simulink library "Lidar_IdealWind_16b"  (Simulink 8.8)
settings: Solver=VariableStepAuto  StartTime=0.0  StopTime=10.0  RelTol=1e-3
undefined symbols (not defined in the file): Atmosphere, CRM, IdealWind, LIDAR, SimConfig, WindReconstruction
libraries: simulink x1
settings Model: SuppressorTable="22 serialization::archive 15 0 6 0 0 1 8 0 0 0 0 6 0 0 1 0 93 Lidar_IdealWind_16b/Lidar_IdealWind/TriggerEstimation/Repeating Sequence Stair/LimitedCounter 0 6 0 0 2 8 0 0 0 0 6 41 Simulink:DataType:WarningOverFlowDetected 0 0 0 6 0  0  0 0 0 0 8 20160608 0 0 0 15 23 17 0 1 40 SimulinkFixedPoint:util:Overflowoccurred 0 0 0  0  8 20160608 0 15 23 17 0 1"  Creator=cava_da  LastModifiedBy=cava_da

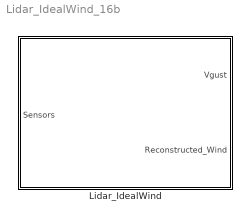
== system Lidar_IdealWind_16b ==
  Lidar_IdealWind : Subsystem

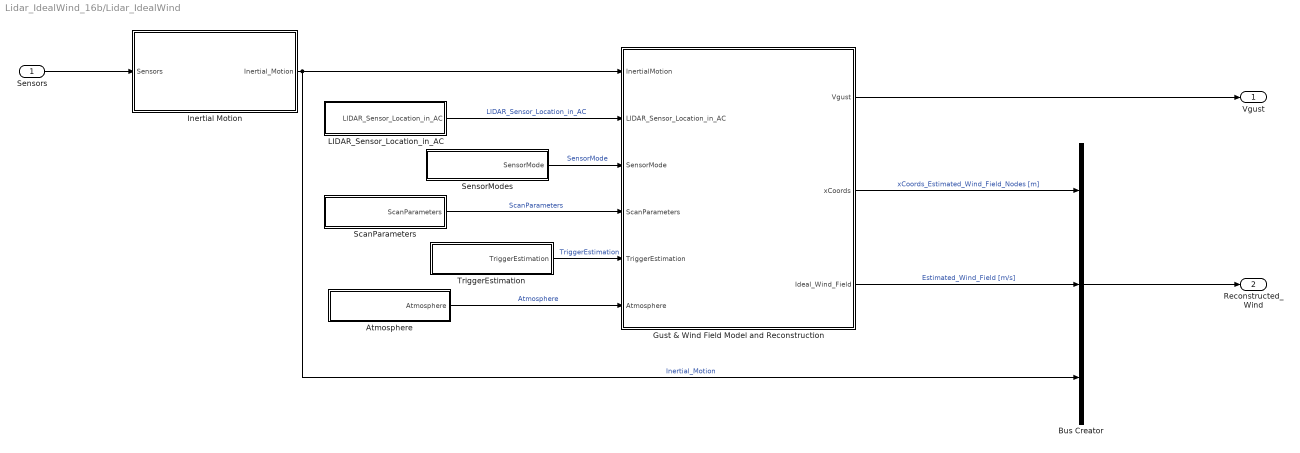
== system Lidar_IdealWind_16b/Lidar_IdealWind ==
  Sensors : Inport
  Atmosphere : Subsystem
  Bus Creator : BusCreator  Inputs=3
  Gust & Wind Field Model and Reconstruction : Subsystem
  Inertial Motion : Subsystem
  LIDAR_Sensor_Location_in_AC : Subsystem
  ScanParameters : Subsystem
  SensorModes : Subsystem
  TriggerEstimation : Subsystem
  Vgust : Outport
  Reconstructed_Wind : Outport  Port=2
  wires:
  Bus Creator/1 -> Reconstructed_Wind/1
  Atmosphere/1(Atmosphere) -> Gust & Wind Field Model and Reconstruction/6(Atmosphere)  "Atmosphere"
  Gust & Wind Field Model and Reconstruction/1(Vgust) -> Vgust/1
  Gust & Wind Field Model and Reconstruction/3(Ideal_Wind_Field) -> Bus Creator/2  "Estimated_Wind_Field [m/s]"
  Gust & Wind Field Model and Reconstruction/2(xCoords) -> Bus Creator/1  "xCoords_Estimated_Wind_Field_Nodes [m]"
  Inertial Motion/1(Inertial_Motion) -> Gust & Wind Field Model and Reconstruction/1(InertialMotion), Bus Creator/3  "Inertial_Motion"
  TriggerEstimation/1(TriggerEstimation) -> Gust & Wind Field Model and Reconstruction/5(TriggerEstimation)  "TriggerEstimation"
  ScanParameters/1(ScanParameters) -> Gust & Wind Field Model and Reconstruction/4(ScanParameters)  "ScanParameters"
  SensorModes/1(SensorMode) -> Gust & Wind Field Model and Reconstruction/3(SensorMode)  "SensorMode"
  LIDAR_Sensor_Location_in_AC/1(LIDAR_Sensor_Location_in_AC) -> Gust & Wind Field Model and Reconstruction/2(LIDAR_Sensor_Location_in_AC)  "LIDAR_Sensor_Location_in_AC"
  Sensors/1 -> Inertial Motion/1(Sensors)

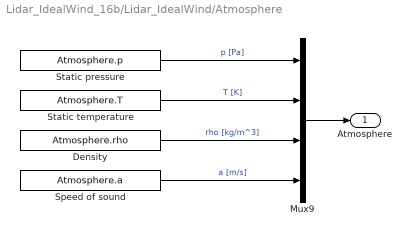
== system Lidar_IdealWind_16b/Lidar_IdealWind/Atmosphere ==
  Density : Constant  Value=Atmosphere.rho
  Mux9 : Mux
  Speed of sound : Constant  Value=Atmosphere.a
  Static pressure : Constant  Value=Atmosphere.p
  Static temperature : Constant  Value=Atmosphere.T
  Atmosphere : Outport
  wires:
  Speed of sound/1 -> Mux9/4  "a [m/s]"
  Density/1 -> Mux9/3  "rho [kg/m^3]"
  Static temperature/1 -> Mux9/2  "T [K]"
  Static pressure/1 -> Mux9/1  "p [Pa]"
  Mux9/1 -> Atmosphere/1

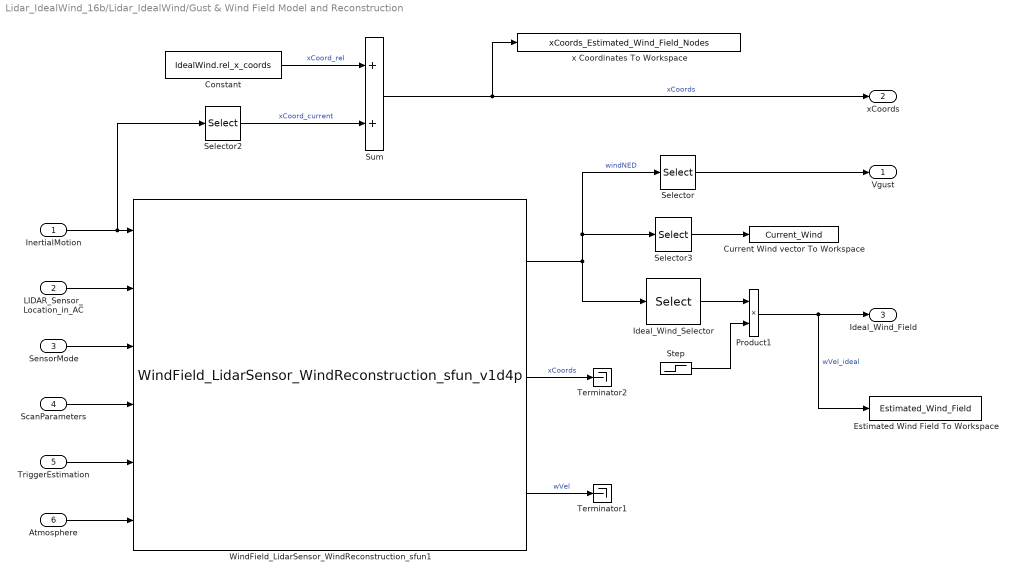
== system Lidar_IdealWind_16b/Lidar_IdealWind/Gust & Wind Field Model and Reconstruction ==
  InertialMotion : Inport
  LIDAR_Sensor_Location_in_AC : Inport  Port=2
  SensorMode : Inport  Port=3
  ScanParameters : Inport  Port=4
  TriggerEstimation : Inport  Port=5
  Atmosphere : Inport  Port=6
  Constant : Constant  Value=IdealWind.rel_x_coords
  Current Wind vector To Workspace : ToWorkspace  VariableName=Current_Wind  SaveFormat=Structure  SampleTime=-1
  Estimated Wind Field To Workspace : ToWorkspace  VariableName=Estimated_Wind_Field  SaveFormat=Structure With Time  SampleTime=-1
      settings: Decimation=SimConfig.Logging.DecimationFactor
  Ideal_Wind_Selector : Selector  IndexOptions=Starting index (dialog)  Indices=4  OutputSizes=IdealWind.n_nodes
  Product1 : Product  RndMeth=Zero
  Selector : Selector  IndexOptions=Index vector (dialog)  Indices=3  OutputSizes=1
  Selector2 : Selector  IndexOptions=Index vector (dialog)  Indices=1  OutputSizes=1
  Selector3 : Selector  IndexOptions=Index vector (dialog)  Indices=1:3  OutputSizes=1
  Step : Step  Time=WindReconstruction.StartEstimationTime  SampleTime=0
  Sum : Sum
  Terminator1 : Terminator
  Terminator2 : Terminator
  WindField_LidarSensor_WindReconstruction_sfun1 : S-Function  FunctionName=WindField_LidarSensor_WindReconstruction_sfun_v1d4p  Parameters=Atmosphere,LIDAR,WindReconstruction  SFunctionDeploymentMode=off  EnableBusSupport=off  mask(Direct detection wind lidar and wind reconstruction (s-function)){}
      mask help:
      | This s-function incorporates the model of a direct detection Doppler wind lidar coupled with a wind reconstruction algorithm based on maximum likelihood estimation. It also serves as the interface between the included wind model and the encompassing aeroelastic aircraft model via the configurable wind output (output port 1).
      | The lidar model and the wind reconstruction algorithm are technically independent modules, but are implemented in the same s-function for performance reasons.
      |
      | Output port 1: wind output, configurable via the parameter Atmosphere.WindConfig
      | Output port 2: x-coordinates of the estimation nodes in geodetic frame and in meters
      | Output port 3: vertical wind speed at the estimation nodes in m/s
      |
      | Output ports 2 and 3 are only updated when a new estimation was triggered via input port 5.
      |
      | Detailed documentation is found under: https://github.com/dlr-ft-gla/GLA-Benchmark/wiki
      |
      |
      |
      | (c) Copyright 2021 DLR e. V.
      |
      | Institute of Flight Systems, 38108 Braunschweig, Germany.
      | Institute of Atmospheric Physics, 82234 Wessling, Germany.
      |
      | Authors:
      | Daniel Kiehn (daniel.kiehn@dlr.de)
      | Nicolas Fezans (nicolas.fezans@dlr.de)
      | Patrick Vrancken (patrick.vrancken@dlr.de)
      |
      | Block and underlying s-function released under CC-BY-ND 4.0 license.
      | https://creativecommons.org/licenses/by-nd/4.0/
      mask Help: For help, please refer to the online documentation of the CRM benchmark model: <a href="matlab: web('https://github.com/dlr-ft-gla/GLA-Benchmark/wiki')">https://github.com/dlr-ft-gla/GLA-Benchmark/wiki</a>.
      mask Display:
      | port_label('input', 1, 'Inertial motion');
      | port_label('input', 2, 'Sensor location in AC');
      | port_label('input', 3, 'Sensor mode');
      | port_label('input', 4, 'Scan parameters');
      | port_label('input', 5, 'Estimation trigger');
      | port_label('input', 6, 'Atmosphere');
      | 
      | port_label('output', 1, 'AC wind inputs');
      | port_label('output', 2, 'x coordinates');
      | port_label('output', 3, 'Estimated wind');
      | 
      | image(imread('DLR_Logo.jpg'),[180,10,81,68])
      | 
      | disp(['DIRECT DETECTION WIND LIDAR\n',...
      | '& WIND RECONSTRUCTION ALGORITHM\n\n\n\n',...
      | '(c) Copyright 2021 DLR e. V.\n\n',...
      | 'Institute of Flight Systems\n',...
      | 'Institute of Atmospheric Physics\n\n',...
      | 'Authors:\n',...
      | 'Daniel Kiehn (daniel.kiehn@dlr.de)\n',...
      | 'Nicolas Fezans (nicolas.fezans@dlr.de)\n',...
      | 'Patrick Vrancken (patrick.vrancken@dlr.de)\n\n\n',...
      | 'Block and underlying s-function\n',...
      | 'released under CC-BY-ND 4.0 license.'])
  x Coordinates To Workspace : ToWorkspace  VariableName=xCoords_Estimated_Wind_Field_Nodes  SaveFormat=Structure With Time  SampleTime=-1
      settings: Decimation=SimConfig.Logging.DecimationFactor
  Vgust : Outport
  xCoords : Outport  Port=2
  Ideal_Wind_Field : Outport  Port=3
  wires:
  Atmosphere/1 -> WindField_LidarSensor_WindReconstruction_sfun1/6
  Selector/1 -> Vgust/1
  TriggerEstimation/1 -> WindField_LidarSensor_WindReconstruction_sfun1/5
  ScanParameters/1 -> WindField_LidarSensor_WindReconstruction_sfun1/4
  SensorMode/1 -> WindField_LidarSensor_WindReconstruction_sfun1/3
  LIDAR_Sensor_Location_in_AC/1 -> WindField_LidarSensor_WindReconstruction_sfun1/2
  InertialMotion/1 -> Selector2/1, WindField_LidarSensor_WindReconstruction_sfun1/1
  WindField_LidarSensor_WindReconstruction_sfun1/2 -> Terminator2/1  "xCoords"
  WindField_LidarSensor_WindReconstruction_sfun1/3 -> Terminator1/1  "wVel"
  Selector2/1 -> Sum/2  "xCoord_current"
  Constant/1 -> Sum/1  "xCoord_rel"
  Sum/1 -> x Coordinates To Workspace/1, xCoords/1  "xCoords"
  Selector3/1 -> Current Wind vector To Workspace/1
  WindField_LidarSensor_WindReconstruction_sfun1/1 -> Selector3/1, Selector/1, Ideal_Wind_Selector/1  "windNED"
  Step/1 -> Product1/2
  Ideal_Wind_Selector/1 -> Product1/1
  Product1/1 -> Estimated Wind Field To Workspace/1, Ideal_Wind_Field/1  "wVel_ideal"

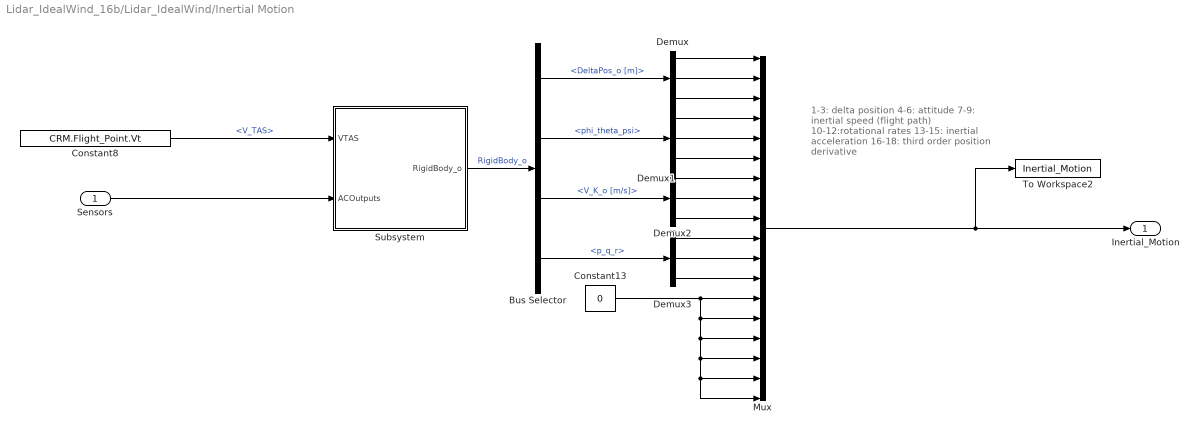
== system Lidar_IdealWind_16b/Lidar_IdealWind/Inertial Motion ==
  note: 1-3: delta position
      | 4-6: attitude
      | 7-9: inertial speed (flight path)
      | 10-12:rotational rates
      | 13-15: inertial acceleration
      | 16-18: third order position derivative
  Sensors : Inport
  Bus Selector : BusSelector  OutputSignals=DeltaPos_o [m],phi_theta_psi,V_K_o [m/s],p_q_r
  Constant13 : Constant  Value=0
  Constant8 : Constant  Value=CRM.Flight_Point.Vt
  Demux{,1..3} (4 alike) : Demux  Outputs=3
  Mux : Mux  Inputs=18
  Subsystem : Subsystem
  To Workspace2 : ToWorkspace  VariableName=Inertial_Motion  SaveFormat=Structure  SampleTime=-1
      settings: Decimation=SimConfig.Logging.DecimationFactor
  Inertial_Motion : Outport
  wires:
  Constant13/1 -> Mux/13, Mux/14, Mux/15, Mux/16, Mux/18, Mux/17
  Mux/1 -> To Workspace2/1, Inertial_Motion/1
  Constant8/1 -> Subsystem/1(VTAS)  "<V_TAS>"
  Subsystem/1(RigidBody_o) -> Bus Selector/1  "RigidBody_o"
  Sensors/1 -> Subsystem/2(ACOutputs)
  Demux3/3 -> Mux/12
  Demux3/2 -> Mux/11
  Demux3/1 -> Mux/10
  Demux2/3 -> Mux/9
  Demux2/2 -> Mux/8
  Demux2/1 -> Mux/7
  Demux1/3 -> Mux/6
  Demux1/2 -> Mux/5
  Demux1/1 -> Mux/4
  Demux/3 -> Mux/3
  Demux/2 -> Mux/2
  Demux/1 -> Mux/1
  Bus Selector/3 -> Demux2/1  "<V_K_o [m/s]>"
  Bus Selector/2 -> Demux1/1  "<phi_theta_psi>"
  Bus Selector/1 -> Demux/1  "<DeltaPos_o [m]>"
  Bus Selector/4 -> Demux3/1  "<p_q_r>"

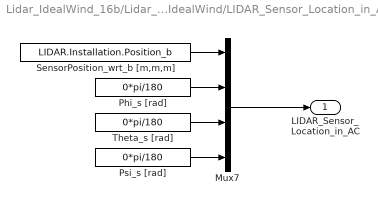
== system Lidar_IdealWind_16b/Lidar_IdealWind/LIDAR_Sensor_Location_in_AC ==
  Mux7 : Mux
  Phi_s [rad] : Constant  Value=0*pi/180
  Psi_s [rad] : Constant  Value=0*pi/180
  SensorPosition_wrt_b [m,m,m] : Constant  Value=LIDAR.Installation.Position_b
  Theta_s [rad] : Constant  Value=0*pi/180
  LIDAR_Sensor_Location_in_AC : Outport
  wires:
  Mux7/1 -> LIDAR_Sensor_Location_in_AC/1
  Psi_s [rad]/1 -> Mux7/4
  Theta_s [rad]/1 -> Mux7/3
  Phi_s [rad]/1 -> Mux7/2
  SensorPosition_wrt_b [m,m,m]/1 -> Mux7/1

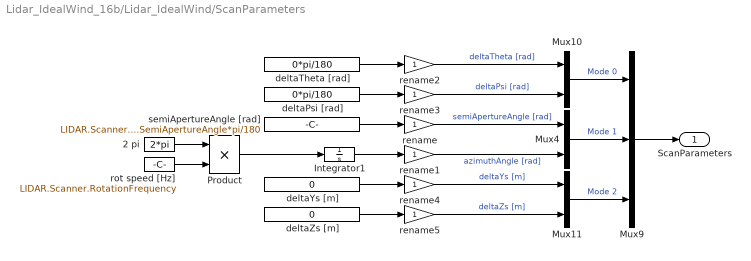
== system Lidar_IdealWind_16b/Lidar_IdealWind/ScanParameters ==
  2 pi : Constant  Value=2*pi
  Integrator1 : Integrator
  Mux10 : Mux  Inputs=2
  Mux11 : Mux  Inputs=2
  Mux4 : Mux  Inputs=2
  Mux9 : Mux  Inputs=3
  Product : Product  RndMeth=Zero
  deltaPsi [rad] : Constant  Value=0*pi/180  OutDataTypeStr=double
  deltaTheta [rad] : Constant  Value=0*pi/180  OutDataTypeStr=double
  deltaYs [m] : Constant  Value=0  OutDataTypeStr=double
  deltaZs [m] : Constant  Value=0  OutDataTypeStr=double
  rename{,1..5} (6 alike) : Gain
  rot speed [Hz] : Constant  Value=LIDAR.Scanner.RotationFrequency
  semiApertureAngle [rad] : Constant  Value=LIDAR.Scanner.SemiApertureAngle*pi/180  OutDataTypeStr=double
  ScanParameters : Outport
  wires:
  Mux9/1 -> ScanParameters/1
  Integrator1/1 -> rename1/1
  rot speed [Hz]/1 -> Product/2
  Product/1 -> Integrator1/1
  2 pi/1 -> Product/1
  semiApertureAngle [rad]/1 -> rename/1
  deltaZs [m]/1 -> rename5/1
  deltaYs [m]/1 -> rename4/1
  deltaTheta [rad]/1 -> rename2/1
  deltaPsi [rad]/1 -> rename3/1
  Mux11/1 -> Mux9/3  "Mode 2"
  Mux4/1 -> Mux9/2  "Mode 1"
  rename4/1 -> Mux11/1  "deltaYs [m]"
  rename5/1 -> Mux11/2  "deltaZs [m]"
  rename/1 -> Mux4/1  "semiApertureAngle [rad]"
  rename1/1 -> Mux4/2  "azimuthAngle [rad]"
  Mux10/1 -> Mux9/1  "Mode 0"
  rename2/1 -> Mux10/1  "deltaTheta [rad]"
  rename3/1 -> Mux10/2  "deltaPsi [rad]"

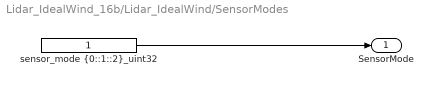
== system Lidar_IdealWind_16b/Lidar_IdealWind/SensorModes ==
  "sensor_mode {0::1::2}_uint32" : Constant  OutDataTypeStr=uint32
  SensorMode : Outport
  wires:
  "sensor_mode {0::1::2}_uint32"/1 -> SensorMode/1

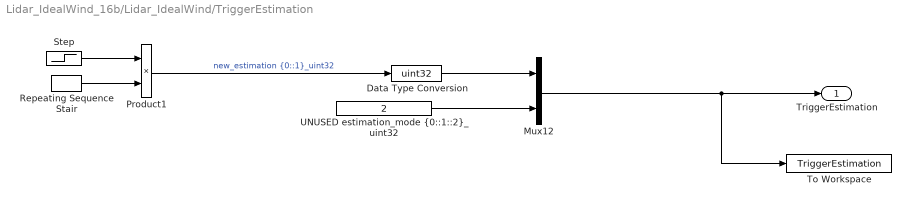
== system Lidar_IdealWind_16b/Lidar_IdealWind/TriggerEstimation ==
  Data Type Conversion : DataTypeConversion  OutDataTypeStr=uint32
  Mux12 : Mux  Inputs=2
  Product1 : Product  RndMeth=Zero
  Repeating Sequence Stair : simulink/Sources/Repeating Sequence Stair  OutValues=[0 zeros(1,(1/(10*SimConfig.SampleTime))-1)].'  tsamp=-1  OutMin=[]  OutMax=[]  OutDataTypeStr=float('double')  OutputDataTypeScalingMode=Specify via dialog  OutDataType=float('double')  ConRadixGroup=Best Precision: Vector-wise  OutScaling=2^-12
  Step : Step  Time=WindReconstruction.StartEstimationTime  SampleTime=0
  To Workspace : ToWorkspace  VariableName=TriggerEstimation  SaveFormat=Structure  SampleTime=-1
  "UNUSED estimation_mode {0::1::2}_uint32" : Constant  Value=2  OutDataTypeStr=uint32
  TriggerEstimation : Outport
  wires:
  Mux12/1 -> To Workspace/1, TriggerEstimation/1
  Step/1 -> Product1/1
  Repeating Sequence Stair/1 -> Product1/2
  Data Type Conversion/1 -> Mux12/1
  "UNUSED estimation_mode {0::1::2}_uint32"/1 -> Mux12/2
  Product1/1 -> Data Type Conversion/1  "new_estimation {0::1}_uint32"

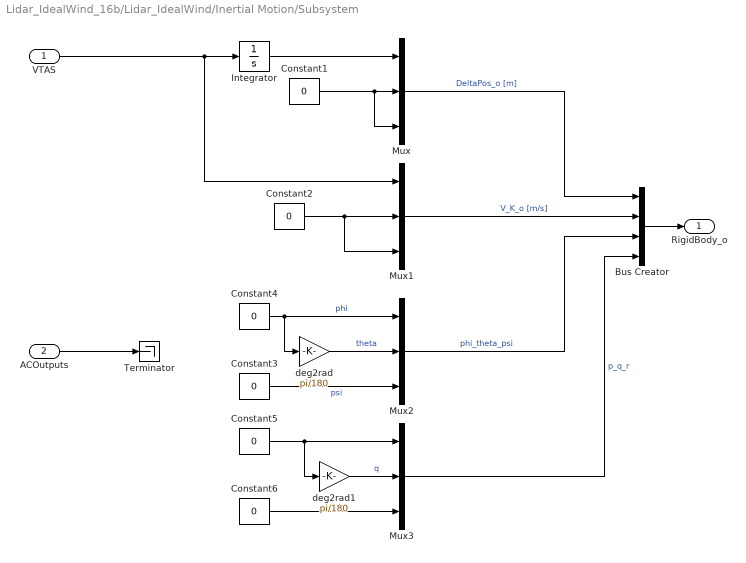
== system Lidar_IdealWind_16b/Lidar_IdealWind/Inertial Motion/Subsystem ==
  VTAS : Inport
  ACOutputs : Inport  Port=2
  Bus Creator : BusCreator  Inputs=4
  Constant{1..6} (6 alike) : Constant  Value=0
  Integrator : Integrator
  Mux{,1..3} (4 alike) : Mux  Inputs=3
  Terminator : Terminator
  deg2rad : Gain  Gain=pi/180
  deg2rad1 : Gain  Gain=pi/180
  RigidBody_o : Outport
  wires:
  ACOutputs/1 -> Terminator/1
  VTAS/1 -> Integrator/1, Mux1/1
  Constant6/1 -> Mux3/3
  Constant5/1 -> deg2rad1/1, Mux3/1
  deg2rad1/1 -> Mux3/2  "q"
  Mux3/1 -> Bus Creator/4  "p_q_r"
  Constant3/1 -> Mux2/3  "psi"
  deg2rad/1 -> Mux2/2  "theta"
  Constant4/1 -> deg2rad/1, Mux2/1  "phi"
  Mux2/1 -> Bus Creator/3  "phi_theta_psi"
  Constant2/1 -> Mux1/3, Mux1/2
  Mux1/1 -> Bus Creator/2  "V_K_o [m/s]"
  Bus Creator/1 -> RigidBody_o/1
  Mux/1 -> Bus Creator/1  "DeltaPos_o [m]"
  Integrator/1 -> Mux/1
  Constant1/1 -> Mux/3, Mux/2
